simulink model "saddle"  (Simulink 6.3)
settings: Solver=ode45  StartTime=0.0  StopTime=10.0  RelTol=1e-3
undefined symbols (not defined in the file or in its folder): k_stable, k_unstable
settings Model: Creator=rana  LastModifiedBy=rana  ExtModeAutoUpdateStatusClock=off

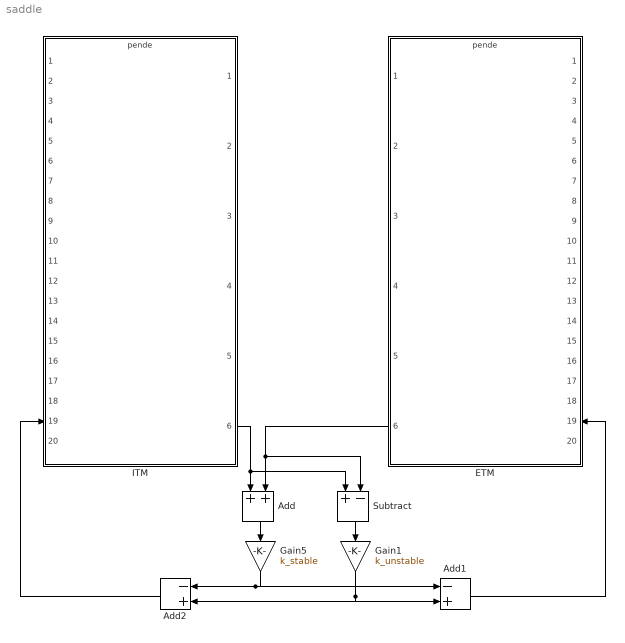
== system saddle ==
  Add : Sum  Orientation=down  OutScaling=2^-10
  Add1 : Sum  Inputs=-+  OutScaling=2^-10
  Add2 : Sum  Orientation=left  Inputs=-+  OutScaling=2^-10
  ETM : ModelReference  Orientation=left  ModelName=pende  ModelReferenceVersion=1.177  CopyOfModelName=pende
  Gain1 : Gain  Orientation=down  Gain=k_unstable
  Gain5 : Gain  Orientation=down  Gain=k_stable
  ITM : ModelReference  ModelName=pende  ModelReferenceVersion=1.177  CopyOfModelName=pende
  Subtract : Sum  Orientation=down  Inputs=+-  OutScaling=2^-10
  wires:
  ITM/6 -> Add/1, Subtract/1
  ETM/6 -> Add/2, Subtract/2
  Add/1 -> Gain5/1
  Subtract/1 -> Gain1/1
  Gain5/1 -> Add2/1, Add1/1
  Add2/1 -> ITM/19
  Gain1/1 -> Add2/2, Add1/2
  Add1/1 -> ETM/19
